simulink library "util_fsw_frame_rotation_lib"  (R2015b)
settings: Solver=ode45  SolverMode=SingleTasking  StartTime=0.0  StopTime=10.0  RelTol=1e-3
values from neighbouring files (symbols this model uses):
  de_cos_coeff = [ 1.5419 ... (first row only)    [util_frame_rotation_init.m]
  de_t_poly = fliplr( [66.5392 +0.0130] )    [util_frame_rotation_init.m]
  e10coeff = fliplr([ 15.134 -0.1589763])    [util_frame_rotation_init.m]
  e11coeff = fliplr([119.743 +0.0036096])    [util_frame_rotation_init.m]
  e12coeff = fliplr([239.961 +0.1643573])    [util_frame_rotation_init.m]
  e13coeff = fliplr([ 25.053 +12.9590088])    [util_frame_rotation_init.m]
  e1coeff = fliplr([125.045 -0.0529921])    [util_frame_rotation_init.m]
  e2coeff = fliplr([250.089 -0.1059842])    [util_frame_rotation_init.m]
  e3coeff = fliplr([260.008 +13.0120009])    [util_frame_rotation_init.m]
  e4coeff = fliplr([176.625 +13.3407154])    [util_frame_rotation_init.m]
  e5coeff = fliplr([357.529 +0.9856003])    [util_frame_rotation_init.m]
  e6coeff = fliplr([311.589 +26.4057084])    [util_frame_rotation_init.m]
  e7coeff = fliplr([134.963 +13.0649930])    [util_frame_rotation_init.m]
  e8coeff = fliplr([276.617 +0.3287146])    [util_frame_rotation_init.m]
  e9coeff = fliplr([ 34.226 +1.7484877])    [util_frame_rotation_init.m]
  omega_moon_iau_coeff = [  3.5610 ... (first row only)    [util_frame_rotation_init.m]
  omega_pa_mat_init = [0 0 0; 0 0 0; 0 0 1]    [util_frame_rotation_init.m]
  ra_sin_coeff = [ -3.8787 ... (first row only)    [util_frame_rotation_init.m]
  ra_t_poly = fliplr( [269.9949 +0.0031] )    [util_frame_rotation_init.m]
undefined symbols (not defined in the file or in its folder): central_body_omega_dot, earth_moon_rotation_matrix_select, ini_epoch_seconds, ini_hour, ini_minute, ini_moon_rotation_rate, ini_seconds, kfl_quat_mcmf_to_topo, kfl_target_site_planet_fixed
libraries: util_quat_lib x67, util_common_lib x22, util_info_lib x18, util_fsw_frame_rotation_lib x9, util_extra_lib x1
(part 2 of 2)

== system util_fsw_frame_rotation_lib/vec_topo_to_mcmf ==
  vec_topo : Inport
  q_mcmf_to_topo : Inport  Port=2
  Library Information : util_info_lib/Library Information  owner='NONE'
  quaternion_conjugate q_topo_to_mcmf : util_quat_lib/quaternion_conjugate  SystemSampleTime=-1
  quaternion_frame_transformation v_mcmf : util_quat_lib/quaternion_frame_transformation  SystemSampleTime=-1
  vec_mcmf : Outport
  wires:
  vec_topo/1 -> quaternion_frame_transformation v_mcmf/1
  [q_mcmf_to_topo] -> quaternion_conjugate q_topo_to_mcmf/1
  quaternion_conjugate q_topo_to_mcmf/1 -> quaternion_frame_transformation v_mcmf/2
  quaternion_frame_transformation v_mcmf/1 -> vec_mcmf/1  "Vector MCMF"
  q_mcmf_to_topo/1 -> [q_mcmf_to_topo]

== system util_fsw_frame_rotation_lib/vector_j2000_to_mcmf ==
  vec_j2000 : Inport
  q_j2000_to_mcmf : Inport  Port=2
  Library Information : util_info_lib/Library Information  owner='NONE'
  quaternion_frame_transformation : util_quat_lib/quaternion_frame_transformation  SystemSampleTime=-1
  vec_mcmf : Outport
  wires:
  quaternion_frame_transformation/1 -> vec_mcmf/1
  vec_j2000/1 -> quaternion_frame_transformation/1
  q_j2000_to_mcmf/1 -> [q_j2000_to_mcmf]
  [q_j2000_to_mcmf] -> quaternion_frame_transformation/2

== system util_fsw_frame_rotation_lib/vector_mcmf_to_j2000 ==
  vec_mcmf : Inport
  q_j2000_to_mcmf : Inport  Port=2
  Library Information : util_info_lib/Library Information  owner='NONE'
  quaternion_conjugate : util_quat_lib/quaternion_conjugate  SystemSampleTime=-1
  quaternion_frame_transformation : util_quat_lib/quaternion_frame_transformation  SystemSampleTime=-1
  vec_j2000 : Outport
  wires:
  vec_mcmf/1 -> quaternion_frame_transformation/1
  quaternion_frame_transformation/1 -> vec_j2000/1
  [q_j2000_to_mcmf] -> quaternion_conjugate/1
  quaternion_conjugate/1 -> quaternion_frame_transformation/2
  q_j2000_to_mcmf/1 -> [q_j2000_to_mcmf]

== system util_fsw_frame_rotation_lib/vector_mcmf_to_topo ==
  vec_mcmf : Inport
  q_mcmf_to_topo : Inport  Port=2
  Library Information : util_info_lib/Library Information  owner='NONE'
  quaternion_frame_transformation1 : util_quat_lib/quaternion_frame_transformation  SystemSampleTime=-1
  vec_topo : Outport
  wires:
  vec_mcmf/1 -> quaternion_frame_transformation1/1
  q_mcmf_to_topo/1 -> [q_mcmf_to_topo]
  quaternion_frame_transformation1/1 -> vec_topo/1
  [q_mcmf_to_topo] -> quaternion_frame_transformation1/2

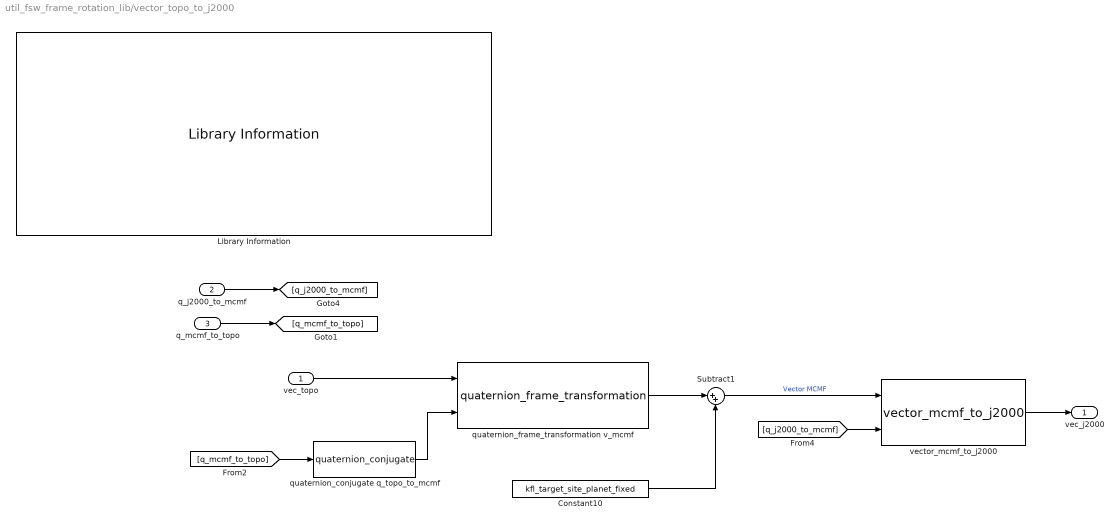
== system util_fsw_frame_rotation_lib/vector_topo_to_j2000 ==
  vec_topo : Inport
  q_j2000_to_mcmf : Inport  Port=2
  q_mcmf_to_topo : Inport  Port=3
  Constant10 : Constant  Value=kfl_target_site_planet_fixed
  Library Information : util_info_lib/Library Information  owner='NONE'
  Subtract1 : Sum  Inputs=|++
  quaternion_conjugate q_topo_to_mcmf : util_quat_lib/quaternion_conjugate  SystemSampleTime=-1
  quaternion_frame_transformation v_mcmf : util_quat_lib/quaternion_frame_transformation  SystemSampleTime=-1
  vector_mcmf_to_j2000 : util_fsw_frame_rotation_lib/vector_mcmf_to_j2000  SystemSampleTime=-1
  vec_j2000 : Outport
  wires:
  vec_topo/1 -> quaternion_frame_transformation v_mcmf/1
  [q_mcmf_to_topo] -> quaternion_conjugate q_topo_to_mcmf/1
  quaternion_conjugate q_topo_to_mcmf/1 -> quaternion_frame_transformation v_mcmf/2
  vector_mcmf_to_j2000/1 -> vec_j2000/1
  Subtract1/1 -> vector_mcmf_to_j2000/1  "Vector MCMF"
  q_mcmf_to_topo/1 -> [q_mcmf_to_topo]
  q_j2000_to_mcmf/1 -> [q_j2000_to_mcmf]
  [q_j2000_to_mcmf] -> vector_mcmf_to_j2000/2
  quaternion_frame_transformation v_mcmf/1 -> Subtract1/1
  Constant10/1 -> Subtract1/2

== system util_fsw_frame_rotation_lib/velocity_j2000_to_mcmf ==
  pos_j2000 : Inport
  vel_j2000 : Inport  Port=2
  q_j2000_to_MCMF : Inport  Port=3
  Add1 : Sum
  Library Information : util_info_lib/Library Information  owner='NONE'
  Moon Rotation Rate : Constant  Value=-ini_moon_rotation_rate
  cross_product Kinematic Term in Moon Rotating Frame : util_common_lib/cross_product  SystemSampleTime=-1
  quaternion_conjugate : util_quat_lib/quaternion_conjugate  SystemSampleTime=-1
  quaternion_frame_transformation : util_quat_lib/quaternion_frame_transformation  SystemSampleTime=-1
  quaternion_frame_transformation1 : util_quat_lib/quaternion_frame_transformation  SystemSampleTime=-1
  quaternion_frame_transformation2 : util_quat_lib/quaternion_frame_transformation  SystemSampleTime=-1
  vel_mcmf : Outport
  wires:
  vel_j2000/1 -> quaternion_frame_transformation/1
  q_j2000_to_MCMF/1 -> quaternion_frame_transformation2/2, quaternion_frame_transformation/2, quaternion_conjugate/1
  Moon Rotation Rate/1 -> quaternion_frame_transformation1/1
  quaternion_conjugate/1 -> quaternion_frame_transformation1/2
  Add1/1 -> vel_mcmf/1
  quaternion_frame_transformation/1 -> Add1/2
  pos_j2000/1 -> cross_product Kinematic Term in Moon Rotating Frame/2
  quaternion_frame_transformation2/1 -> Add1/1
  cross_product Kinematic Term in Moon Rotating Frame/1 -> quaternion_frame_transformation2/1
  quaternion_frame_transformation1/1 -> cross_product Kinematic Term in Moon Rotating Frame/1  "Negative Sense Moon rotation vector in J2000"

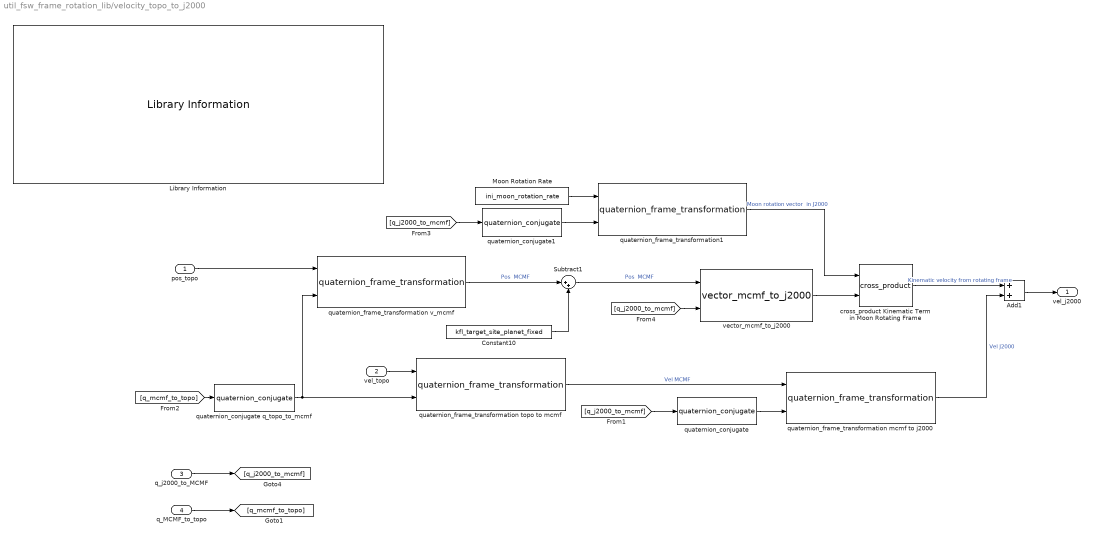
== system util_fsw_frame_rotation_lib/velocity_topo_to_j2000 ==
  pos_topo : Inport
  vel_topo : Inport  Port=2
  q_j2000_to_MCMF : Inport  Port=3
  q_MCMF_to_topo : Inport  Port=4
  Add1 : Sum
  Constant10 : Constant  Value=kfl_target_site_planet_fixed
  Library Information : util_info_lib/Library Information  owner='NONE'
  Moon Rotation Rate : Constant  Value=ini_moon_rotation_rate
  Subtract1 : Sum  Inputs=|++
  cross_product Kinematic Term in Moon Rotating Frame : util_common_lib/cross_product  SystemSampleTime=-1
  quaternion_conjugate : util_quat_lib/quaternion_conjugate  SystemSampleTime=-1
  quaternion_conjugate q_topo_to_mcmf : util_quat_lib/quaternion_conjugate  SystemSampleTime=-1
  quaternion_conjugate1 : util_quat_lib/quaternion_conjugate  SystemSampleTime=-1
  quaternion_frame_transformation mcmf to j2000 : util_quat_lib/quaternion_frame_transformation  SystemSampleTime=-1
  quaternion_frame_transformation topo to mcmf : util_quat_lib/quaternion_frame_transformation  SystemSampleTime=-1
  quaternion_frame_transformation v_mcmf : util_quat_lib/quaternion_frame_transformation  SystemSampleTime=-1
  quaternion_frame_transformation1 : util_quat_lib/quaternion_frame_transformation  SystemSampleTime=-1
  vector_mcmf_to_j2000 : util_fsw_frame_rotation_lib/vector_mcmf_to_j2000  SystemSampleTime=-1
  vel_j2000 : Outport
  wires:
  pos_topo/1 -> quaternion_frame_transformation v_mcmf/1
  [q_mcmf_to_topo] -> quaternion_conjugate q_topo_to_mcmf/1
  quaternion_conjugate q_topo_to_mcmf/1 -> quaternion_frame_transformation v_mcmf/2, quaternion_frame_transformation topo to mcmf/2
  Subtract1/1 -> vector_mcmf_to_j2000/1  "Pos  MCMF"
  vel_topo/1 -> quaternion_frame_transformation topo to mcmf/1
  quaternion_frame_transformation topo to mcmf/1 -> quaternion_frame_transformation mcmf to j2000/1  "Vel MCMF"
  Moon Rotation Rate/1 -> quaternion_frame_transformation1/1
  quaternion_frame_transformation1/1 -> cross_product Kinematic Term in Moon Rotating Frame/1  "Moon rotation vector  in J2000"
  vector_mcmf_to_j2000/1 -> cross_product Kinematic Term in Moon Rotating Frame/2
  Add1/1 -> vel_j2000/1
  quaternion_frame_transformation mcmf to j2000/1 -> Add1/2  "Vel J2000"
  cross_product Kinematic Term in Moon Rotating Frame/1 -> Add1/1  "Kinematic velocity from rotating frame"
  quaternion_conjugate/1 -> quaternion_frame_transformation mcmf to j2000/2
  q_MCMF_to_topo/1 -> [q_mcmf_to_topo]
  q_j2000_to_MCMF/1 -> [q_j2000_to_mcmf]
  [q_j2000_to_mcmf] -> vector_mcmf_to_j2000/2
  [q_j2000_to_mcmf] -> quaternion_conjugate/1
  [q_j2000_to_mcmf] -> quaternion_conjugate1/1
  quaternion_conjugate1/1 -> quaternion_frame_transformation1/2
  quaternion_frame_transformation v_mcmf/1 -> Subtract1/1  "Pos  MCMF"
  Constant10/1 -> Subtract1/2
